simulink model "myModel"  (R2020a)
settings: Solver=VariableStepAuto  StartTime=0.0  StopTime=30  RelTol=1e-3
undefined symbols (not defined in the file): ampl
libraries: cstblocks x2
settings Model: NumberOfSteps=10  SnapshotBufferSize=50  SnapshotInterval=50  Creator=Strel  LastModifiedBy=Strel
settings DataIOCC: SaveFinalState=on  SaveState=on
settings DebuggingCC: ArithmeticOperatorsInVariantConditions=warning
settings SFSimCC: SimUseLocalCustomCode=off  CustomCodeUndefinedFunction=UseInterfaceOnly
settings RTWCC: RTWUseLocalCustomCode=off

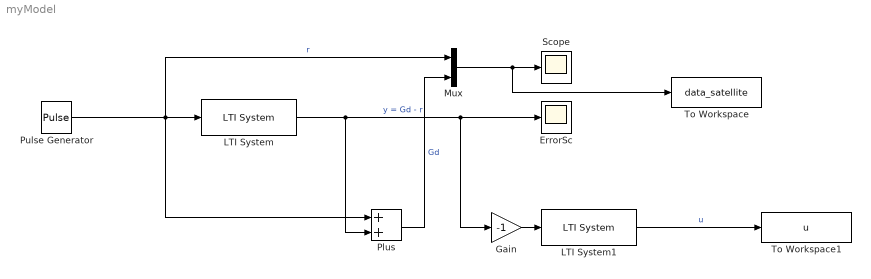
== system myModel ==
  ErrorSc : Scope
  Gain : Gain  Gain=-1
  LTI System : cstblocks/LTI System  sys=P_star_K  IC=[]
  LTI System1 : cstblocks/LTI System  sys=Kd  IC=[]
  Mux : Mux  Inputs=2
  Plus : Sum
  Pulse Generator : DiscretePulseGenerator  PulseType=Time based  Amplitude=ampl  Period=10  PulseWidth=50
  Scope : Scope
  To Workspace : ToWorkspace  VariableName=data_satellite  SaveFormat=Timeseries  SampleTime=-1
  To Workspace1 : ToWorkspace  VariableName=u  SaveFormat=Timeseries  SampleTime=-1
  wires:
  Pulse Generator/1 -> Mux/1, Plus/1, LTI System/1  "r"
  LTI System/1 -> Plus/2, Gain/1, ErrorSc/1  "y = Gd - r"
  Mux/1 -> To Workspace/1, Scope/1
  Plus/1 -> Mux/2  "Gd"
  Gain/1 -> LTI System1/1
  LTI System1/1 -> To Workspace1/1  "u"
